simulink model "DrivelineTest"  (R2021a)
settings: Solver=VariableStepAuto  StartTime=0.0  StopTime=10.0  RelTol=1e-3
libraries: sdl_lib x5, fl_lib x3, SimscapeFluids_lib x3, nesl_utility x2
settings Model: Creator=home  LastModifiedBy=home

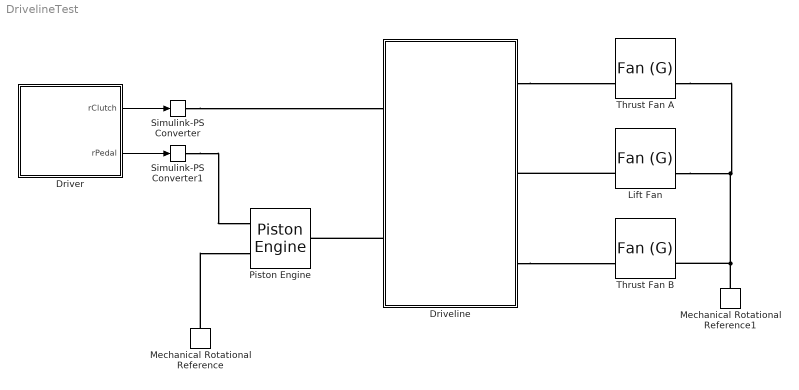
== system DrivelineTest ==
  Driveline : Subsystem
  Driver : Subsystem
  Lift Fan : SimscapeFluids_lib/Gas/Turbomachinery/Fan (G)  fan_spec=fluids.gas.enum.fan_spec.table1D  mech_orientation=simscape.enum.posneg.positive  flow_rate_1D_TLU=[4.7, 5.2, 5.7, 6.1, 6.6] m^3/s  Dp_1D_TLU=[1120, 995.36, 870.94, 746.52, 622.1] Pa  eta_1D_TLU=[.1, .2, .25, .15, .1]  rho_ref_1D=1.2 kg/m^3  omega_ref_1D=910 rpm  omega_Dp_TLU=[450, 500, 550, 600, 650] rpm  flow_rate_Dp_TLU=[.2, .3, .4, .5] m^3/s  Dp_TLU=[675, 650, 560, 420; 830, 800, 695, 520; 1008, 966, 840, 630; 1200, 1150, 1000, 750; 1370, 1300, 1250, 1000] Pa  eta_Dp_TLU=[.22, .23, .25, .24; .38, .39, .4, .34; .58, .6, .62, .6; .81, .82, .84, .8; .88, .91, .95, .9]  omega_flow_TLU=[1800, 2000, 2400, 2800, 3000] rpm  Dp_flow_TLU=[1 / 8, 1 / 4, 3 / 8, 1 / 2] * 3386.4 Pa  flow_rate_TLU=[.3282, .2965, .2556, .1973; .8254, .71, .5876, .4545; 1.2018, 1.0829, .9083, .7034; 1.5065, 1.4098, 1.2722, .9844; 1.8368, 1.7507, 1.6055, 1.2417] m^3/s  eta_flow_TLU=[.22, .23, .25, .24; .38, .39, .4, .34; .58, .6, .62, .6; .81, .82, .84, .8; .88, .91, .95, .9]  omega_DpMax_TLU=[1800, 2000, 2400, 2800, 3000] rpm  DpMax_TLU=[1 / 8, 1 / 4, 3 / 8, 1 / 2, 5 / 8] * 3386.4 Pa  omega_flow_TLU_=[1800, 2000, 2400, 2800, 3000] rpm  Dp_DpMax_TLU=linspace(0, 1, 7)  flow_rate_TLU_=[.3282, .2965, .2556, .1973, .1799, .1288, .0736; .8254, .71, .5876, .4545, .4157, .2967, .1696; 1.2018, 1.0829, .9083, .7034, .6415, .4584, .2619; 1.5065, 1.4098, 1.2722, .9844, .8991, .6418, .3668; 1.8368, 1.7507, 1.6055, 1.2417, 1.1337, .8098, .464] m^3/s  eta_flow_TLU_=[.22, .23, .25, .26, .27, .275, .28; .38, .39, .4, .41, .42, .425, .43; .48, .5, .52, .54, .55, .54, .53; .4, .42, .44, .46, .48, .45, .44; .42, .43, .45, .47, .49, .46, .44]  rho_ref_2D=1.2 kg/m^3  omega_threshold=1 rpm  area_A=0.01 m^2  area_B=0.01 m^2
      settings: SourceProductBaseCode=SH  InternalSimscapePortConfiguration="{\"Bottom\":[],\"Left\":[{\"id\":\"A\",\"label\":\"A\",\"type\":\"foundation.gas.gas\"},{\"id\":\"C\",\"label\":\"C\",\"type\":\"foundation.mechanical.rotational.rotational\"}],\"Right\":[{\"id\":\"B\",\"label\":\"B\",\"type\":\"foundation.gas.gas\"},{\"id\":\"R\",\"label\":\"R\",\"type\":\"foundation.mechanical.rotational.rotational\"}],\"Top\":[]}"
  Mechanical Rotational Reference : fl_lib/Mechanical/Rotational Elements/Mechanical Rotational Reference
  Mechanical Rotational Reference1 : fl_lib/Mechanical/Rotational Elements/Mechanical Rotational Reference
  Piston Engine : sdl_lib/Engines & Motors/Piston Engine  piston_num=4  theta_offset_vector=[0, 180, 360, -180] deg  bore=.10 m  stroke=.06 m  rod=.1 m  stroke_num=4  parameterization=sdl.enum.piston_parameterization.Angle  angle_vector=[-360, -90, -30, 10, 30, 90, 160, 360] deg  throttle_vector=[0, .3, .8, 1]  velocity_vector=[0, 1000, 6000] rpm  pressure_vector=[0, 3, 20, 50, 20, 10, 8, 0] bar  pressure_matrix=[0, 0, 0, 0; 0, .9, 2.4, 3; 0, 6, 16, 20; 0, 15, 40, 50; 0, 6, 16, 20; 0, 3, 8, 10; 0, 2.4, 6.4, 8; 0, 0, 0, 0] bar  pressure_matrix_3D=cat(3, [0, 0, 0, 0; 0, .9, 2.4, 3; 0, 6, 16, 20; 0, 15, 40, 50; 0, 6, 16, 20; 0, 3, 8, 10; 0, 2.4, 6.4, 8; 0, 0, 0, 0], [0, 0, 0, 0; 0, .9, 2.4, 3; 0, 6, 16, 20; 0, 15, 40, 50; 0, 6, 16, 20; 0, 3, 8, 10; 0, 2.4, 6.4, 8; 0, 0, 0, 0], [0, 0, 0, 0; 0, .9, 2.4, 3; 0, 6, 16, 20; 0, 15, 40, 50; 0, 6, 16, 20; 0, 3, 8, 10; 0, 2.4, 6.4, 8; 0, 0, 0, 0]) bar  shaft_dynamics=sdl.enum.shaft_dynamics.On  stiffness=1e6 N*m/rad  damping=1000 N*m/(rad/s)  inertia=.02 kg*m^2  initial_deflection=0 deg  initial_velocity=0 rpm  mu_visc=[0, 0] N*m/(rad/s)  theta_init=90 deg  fc_model=sdl.enum.fuel_consumption_model.FuelOff  fc_per_rev=25 mg/rev  fc_w_tab=[1000, 2000, 3000, 4000, 5000, 6000] rpm  fc_trq_tab=[0, 80, 160, 200, 240, 320, 360, 400] N*m  fc_tab=[.5, .9, 1.4, 1.6, 1.9, 2.7, 3.4, 4.4; 1, 1.7, 2.7, 3.1, 3.6, 5, 6, 7.4; 1.4, 2.7, 4, 4.8, 5.6, 7.5, 8.5, 10.5; 2, 3.6, 5.8, 6.7, 8, 10.4, 11.7, 13.3; 2.5, 4.8, 7.9, 9.4, 10.8, 14, 16.2, 18.6; 3.1, 6, 10.3, 11.9, 13.8, 18.4, 22, 26.5] g/s  bmep_tab=[0, 250, 500, 625, 750, 1000, 1150, 1250] kPa  bsfc_tab=[410, 380, 300, 280, 270, 290, 320, 380; 410, 370, 290, 270, 260, 270, 285, 320; 415, 380, 290, 275, 265, 270, 270, 300; 420, 390, 310, 290, 285, 280, 280, 285; 430, 410, 340, 320, 310, 300, 310, 320; 450, 430, 370, 340, 330, 330, 350, 380] g/hr/kW  fc_interp_method=simscape.enum.interpolation.linear
      settings: SourceProductBaseCode=LD  InternalSimscapePortConfiguration="{\"Bottom\":[],\"Left\":[{\"id\":\"T\",\"label\":\"T\",\"type\":\"input\"},{\"id\":\"B\",\"label\":\"B\",\"type\":\"foundation.mechanical.rotational.rotational\"}],\"Right\":[{\"id\":\"F\",\"label\":\"F\",\"type\":\"foundation.mechanical.rotational.rotational\"}],\"Top\":[]}"
  Simulink-PS Converter : nesl_utility/Simulink-PS Converter  PhysicalDomain=network_engine_domain  SubClassName=ps_input  LeftPortType=input  RightPortType=output  PseudoPeriodic=off  Frequencies=[]  NoiseDistribution=none  NoiseParameters=[]  Unit=1  AffineConversion=off  FilteringAndDerivatives=provide  SimscapeFilterOrder=1  InputFilterTimeConstant=0.001  UdotUserProvided=0
      settings: SourceProductBaseCode=PW,SS
  Simulink-PS Converter1 : nesl_utility/Simulink-PS Converter  PhysicalDomain=network_engine_domain  SubClassName=ps_input  LeftPortType=input  RightPortType=output  PseudoPeriodic=off  Frequencies=[]  NoiseDistribution=none  NoiseParameters=[]  Unit=1  AffineConversion=off  FilteringAndDerivatives=provide  SimscapeFilterOrder=1  InputFilterTimeConstant=0.001  UdotUserProvided=0
      settings: SourceProductBaseCode=PW,SS
  Thrust Fan A : SimscapeFluids_lib/Gas/Turbomachinery/Fan (G)  fan_spec=fluids.gas.enum.fan_spec.table1D  mech_orientation=simscape.enum.posneg.positive  flow_rate_1D_TLU=[4.7, 5.2, 5.7, 6.1, 6.6] m^3/s  Dp_1D_TLU=[1120, 995.36, 870.94, 746.52, 622.1] Pa  eta_1D_TLU=[.1, .2, .25, .15, .1]  rho_ref_1D=1.2 kg/m^3  omega_ref_1D=910 rpm  omega_Dp_TLU=[450, 500, 550, 600, 650] rpm  flow_rate_Dp_TLU=[.2, .3, .4, .5] m^3/s  Dp_TLU=[675, 650, 560, 420; 830, 800, 695, 520; 1008, 966, 840, 630; 1200, 1150, 1000, 750; 1370, 1300, 1250, 1000] Pa  eta_Dp_TLU=[.22, .23, .25, .24; .38, .39, .4, .34; .58, .6, .62, .6; .81, .82, .84, .8; .88, .91, .95, .9]  omega_flow_TLU=[1800, 2000, 2400, 2800, 3000] rpm  Dp_flow_TLU=[1 / 8, 1 / 4, 3 / 8, 1 / 2] * 3386.4 Pa  flow_rate_TLU=[.3282, .2965, .2556, .1973; .8254, .71, .5876, .4545; 1.2018, 1.0829, .9083, .7034; 1.5065, 1.4098, 1.2722, .9844; 1.8368, 1.7507, 1.6055, 1.2417] m^3/s  eta_flow_TLU=[.22, .23, .25, .24; .38, .39, .4, .34; .58, .6, .62, .6; .81, .82, .84, .8; .88, .91, .95, .9]  omega_DpMax_TLU=[1800, 2000, 2400, 2800, 3000] rpm  DpMax_TLU=[1 / 8, 1 / 4, 3 / 8, 1 / 2, 5 / 8] * 3386.4 Pa  omega_flow_TLU_=[1800, 2000, 2400, 2800, 3000] rpm  Dp_DpMax_TLU=linspace(0, 1, 7)  flow_rate_TLU_=[.3282, .2965, .2556, .1973, .1799, .1288, .0736; .8254, .71, .5876, .4545, .4157, .2967, .1696; 1.2018, 1.0829, .9083, .7034, .6415, .4584, .2619; 1.5065, 1.4098, 1.2722, .9844, .8991, .6418, .3668; 1.8368, 1.7507, 1.6055, 1.2417, 1.1337, .8098, .464] m^3/s  eta_flow_TLU_=[.22, .23, .25, .26, .27, .275, .28; .38, .39, .4, .41, .42, .425, .43; .48, .5, .52, .54, .55, .54, .53; .4, .42, .44, .46, .48, .45, .44; .42, .43, .45, .47, .49, .46, .44]  rho_ref_2D=1.2 kg/m^3  omega_threshold=1 rpm  area_A=0.01 m^2  area_B=0.01 m^2
      settings: SourceProductBaseCode=SH  InternalSimscapePortConfiguration="{\"Bottom\":[],\"Left\":[{\"id\":\"A\",\"label\":\"A\",\"type\":\"foundation.gas.gas\"},{\"id\":\"C\",\"label\":\"C\",\"type\":\"foundation.mechanical.rotational.rotational\"}],\"Right\":[{\"id\":\"B\",\"label\":\"B\",\"type\":\"foundation.gas.gas\"},{\"id\":\"R\",\"label\":\"R\",\"type\":\"foundation.mechanical.rotational.rotational\"}],\"Top\":[]}"
  Thrust Fan B : SimscapeFluids_lib/Gas/Turbomachinery/Fan (G)  fan_spec=fluids.gas.enum.fan_spec.table1D  mech_orientation=simscape.enum.posneg.positive  flow_rate_1D_TLU=[4.7, 5.2, 5.7, 6.1, 6.6] m^3/s  Dp_1D_TLU=[1120, 995.36, 870.94, 746.52, 622.1] Pa  eta_1D_TLU=[.1, .2, .25, .15, .1]  rho_ref_1D=1.2 kg/m^3  omega_ref_1D=910 rpm  omega_Dp_TLU=[450, 500, 550, 600, 650] rpm  flow_rate_Dp_TLU=[.2, .3, .4, .5] m^3/s  Dp_TLU=[675, 650, 560, 420; 830, 800, 695, 520; 1008, 966, 840, 630; 1200, 1150, 1000, 750; 1370, 1300, 1250, 1000] Pa  eta_Dp_TLU=[.22, .23, .25, .24; .38, .39, .4, .34; .58, .6, .62, .6; .81, .82, .84, .8; .88, .91, .95, .9]  omega_flow_TLU=[1800, 2000, 2400, 2800, 3000] rpm  Dp_flow_TLU=[1 / 8, 1 / 4, 3 / 8, 1 / 2] * 3386.4 Pa  flow_rate_TLU=[.3282, .2965, .2556, .1973; .8254, .71, .5876, .4545; 1.2018, 1.0829, .9083, .7034; 1.5065, 1.4098, 1.2722, .9844; 1.8368, 1.7507, 1.6055, 1.2417] m^3/s  eta_flow_TLU=[.22, .23, .25, .24; .38, .39, .4, .34; .58, .6, .62, .6; .81, .82, .84, .8; .88, .91, .95, .9]  omega_DpMax_TLU=[1800, 2000, 2400, 2800, 3000] rpm  DpMax_TLU=[1 / 8, 1 / 4, 3 / 8, 1 / 2, 5 / 8] * 3386.4 Pa  omega_flow_TLU_=[1800, 2000, 2400, 2800, 3000] rpm  Dp_DpMax_TLU=linspace(0, 1, 7)  flow_rate_TLU_=[.3282, .2965, .2556, .1973, .1799, .1288, .0736; .8254, .71, .5876, .4545, .4157, .2967, .1696; 1.2018, 1.0829, .9083, .7034, .6415, .4584, .2619; 1.5065, 1.4098, 1.2722, .9844, .8991, .6418, .3668; 1.8368, 1.7507, 1.6055, 1.2417, 1.1337, .8098, .464] m^3/s  eta_flow_TLU_=[.22, .23, .25, .26, .27, .275, .28; .38, .39, .4, .41, .42, .425, .43; .48, .5, .52, .54, .55, .54, .53; .4, .42, .44, .46, .48, .45, .44; .42, .43, .45, .47, .49, .46, .44]  rho_ref_2D=1.2 kg/m^3  omega_threshold=1 rpm  area_A=0.01 m^2  area_B=0.01 m^2
      settings: SourceProductBaseCode=SH  InternalSimscapePortConfiguration="{\"Bottom\":[],\"Left\":[{\"id\":\"A\",\"label\":\"A\",\"type\":\"foundation.gas.gas\"},{\"id\":\"C\",\"label\":\"C\",\"type\":\"foundation.mechanical.rotational.rotational\"}],\"Right\":[{\"id\":\"B\",\"label\":\"B\",\"type\":\"foundation.gas.gas\"},{\"id\":\"R\",\"label\":\"R\",\"type\":\"foundation.mechanical.rotational.rotational\"}],\"Top\":[]}"
  wires:
  Driver/1(rClutch) -> Simulink-PS Converter/1
  Driver/2(rPedal) -> Simulink-PS Converter1/1
  connections:
  Mechanical Rotational Reference/LConn1 -- Piston Engine/LConn2
  Mechanical Rotational Reference1/LConn1 -- Thrust Fan A/RConn2 -- Lift Fan/RConn2 -- Thrust Fan B/RConn2
  Driveline/RConn1 -- Thrust Fan A/LConn2
  Lift Fan/LConn2 -- Driveline/RConn2
  Driveline/LConn2 -- Piston Engine/RConn1
  Driveline/RConn3 -- Thrust Fan B/LConn2
  Simulink-PS Converter/RConn1 -- Driveline/LConn1
  Simulink-PS Converter1/RConn1 -- Piston Engine/LConn1

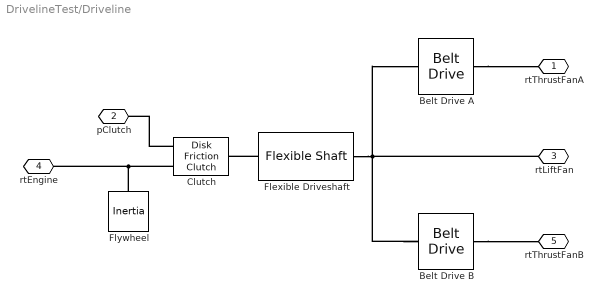
== system DrivelineTest/Driveline ==
  Belt Drive A : sdl_lib/Couplings & Drives/Belt Drive  drive_type=sdl.enum.wrap_configuration.open  belt_type=sdl.enum.belt_type.ideal  sheave_ang=30 deg  num_belts=1  model_f_c=sdl.enum.model_centrifugal.off  linear_density=0.6 kg/m  model_compliance=sdl.enum.compliance.on  stiffness=1e4 N/m  damping=1e3 N/(m/s)  tension=100 N  breakable=sdl.enum.max_tension.off  F_max=1e5 N  r_pulley_A=.15 m  r_pulley_B=.30 m  b_pulley_A=0 N*m/(rad/s)  b_pulley_B=0.001 N*m/(rad/s)  model_inertia_A=sdl.enum.model_inertia.off  model_inertia_B=sdl.enum.model_inertia.off  pulley_inertia_A=0.01 kg*m^2  pulley_inertia_B=0.03 kg*m^2  initial_velocity_A=0 rad/s  initial_velocity_B=0 rad/s  mu=0.5  wrap_parameterization=sdl.enum.wrap_parameterization.centers  d_centers=0.5 m  phi_wrap_A=145 deg  phi_wrap_B=215 deg  v_thr=0.001 m/s
      settings: SourceProductBaseCode=LD  InternalSimscapePortConfiguration="{\"Bottom\":[],\"Left\":[{\"id\":\"A\",\"label\":\"A\",\"type\":\"foundation.mechanical.rotational.rotational\"}],\"Right\":[{\"id\":\"B\",\"label\":\"B\",\"type\":\"foundation.mechanical.rotational.rotational\"}],\"Top\":[]}"
  Belt Drive B : sdl_lib/Couplings & Drives/Belt Drive  drive_type=sdl.enum.wrap_configuration.open  belt_type=sdl.enum.belt_type.ideal  sheave_ang=30 deg  num_belts=1  model_f_c=sdl.enum.model_centrifugal.off  linear_density=0.6 kg/m  model_compliance=sdl.enum.compliance.on  stiffness=1e4 N/m  damping=1e3 N/(m/s)  tension=100 N  breakable=sdl.enum.max_tension.off  F_max=1e5 N  r_pulley_A=.15 m  r_pulley_B=.30 m  b_pulley_A=0 N*m/(rad/s)  b_pulley_B=0.001 N*m/(rad/s)  model_inertia_A=sdl.enum.model_inertia.off  model_inertia_B=sdl.enum.model_inertia.off  pulley_inertia_A=0.01 kg*m^2  pulley_inertia_B=0.03 kg*m^2  initial_velocity_A=0 rad/s  initial_velocity_B=0 rad/s  mu=0.5  wrap_parameterization=sdl.enum.wrap_parameterization.centers  d_centers=0.5 m  phi_wrap_A=145 deg  phi_wrap_B=215 deg  v_thr=0.001 m/s
      settings: SourceProductBaseCode=LD  InternalSimscapePortConfiguration="{\"Bottom\":[],\"Left\":[{\"id\":\"A\",\"label\":\"A\",\"type\":\"foundation.mechanical.rotational.rotational\"}],\"Right\":[{\"id\":\"B\",\"label\":\"B\",\"type\":\"foundation.mechanical.rotational.rotational\"}],\"Top\":[]}"
  Clutch : sdl_lib/Clutches/Disk Friction Clutch  geometry_model=sdl.enum.friction_geometry.radius  r_eff=130 mm  d_o=150 mm  d_i=100 mm  nS=4  piston_area=0.001 m^2  unidirectional=sdl.enum.directionality.bidirectional  friction_model=sdl.enum.friction_model_TLU_thermal.fixed  mu_w_vector=[0, 100, 1000] rad/s  temperature_TLU=[280, 300, 320] K  mu_static=0.35  mu_static_vector=[.4, .38, .36]  mu_coulomb=0.3  mu_coulomb_vector=[.3, .22, .19]  mu_coulomb_temp_vector=[.3, .28, .25]  mu_coulomb_matrix=[.34, .32, .3; .3, .28, .25; .25, .2, .15]  mu_interp_method=simscape.enum.interpolation.linear  mu_extrap_method=simscape.enum.extrapolation.linear  d_f=1  w_tol=0.001 rad/s  pressure_min=100 Pa  mu_visc=0 N*m/(rad/s)  initial_state_locked=sdl.enum.initial_lock.unlocked  enable_faults=simscape.enum.onoff.off  fault_type=sdl.enum.clutchFault.lock  external_fault=simscape.enum.onoff.off  temporal_fault=simscape.enum.onoff.off  fault_time=5 s  report_fault=simscape.enum.assert.action.none  thermal_mass=50 kJ/K  T_init=300 K
      settings: SourceProductBaseCode=LD  InternalSimscapePortConfiguration="{\"Bottom\":[],\"Left\":[{\"id\":\"P\",\"label\":\"P\",\"type\":\"input\"},{\"id\":\"B\",\"label\":\"B\",\"type\":\"foundation.mechanical.rotational.rotational\"}],\"Right\":[{\"id\":\"F\",\"label\":\"F\",\"type\":\"foundation.mechanical.rotational.rotational\"}],\"Top\":[]}"
  Flexible Driveshaft : sdl_lib/Couplings & Drives/Flexible Shaft  modelTransverse=simscape.enum.onoff.off  n_segments=1  parameterization=sdl.enum.shaftParameterization.StiffnessInertia  length=1 m  lengths=[1, .5, .25] m  shaft_stiffness=2e5 N*m/rad  shaft_inertia=0.02 kg*m^2  shaft_stiffnesses=[400000, 200000, 100000] N*m/rad  shaft_inertias=[.025, .02, .015] kg*m^2  eiIN=5e5 m^4*Pa  rhoaIN=19 kg/m  eiINs=[600000, 500000, 400000] m^4*Pa  rhoaINs=[20, 19, 18] kg/m  density=7.8e3 kg/m^3  shear_modulus=7.93e9 Pa  elastic_modulus=200e9 Pa  shaft_construction=sdl.enum.shaftConstruction.solid  diameter_outer=0.075 m  diameter_inner=0.05 m  diameter_outers=[.085, .075, .065] m  diameter_inners=[.055, .05, .045] m  damping_ratio=0.01  mu_visc_BF=[0, 0] N*m/(rad/s)  mu_visc=[0, 0] N*m/(rad/s)  initial_deflection=0 rad  initial_velocity=0 rpm  num_supports=sdl.enum.num_supports.two  z_support=[0, 1] m  boundaryB1=sdl.enum.shaftSupport.clamp  DrotB1_row=[1000, 1000] N*m/(rad/s)  DtransB1_row=[20000, -44000, -44000, 350000] N/(m/s)  DtransB1_w_mat=[20000, -44000, -44000, 350000; 10000, -25000, -25000, 140000; 5000, -10000, -10000, 20000] N/(m/s)  KrotB1_row=[10000, 10000] N*m/rad  KtransB1_row=[1000000, -200000, -300000, 5000000] N/m  KtransB1_w_mat=[1000000, -600000, -3500000, 8000000; 1000000, -200000, -3000000, 5000000; 1000000, -50000, -2500000, 3000000] N/m  boundaryI1=sdl.enum.shaftSupport.clamp  DrotI1_row=[1000, 1000] N*m/(rad/s)  DtransI1_row=[20000, -44000, -44000, 350000] N/(m/s)  DtransI1_w_mat=[20000, -44000, -44000, 350000; 10000, -25000, -25000, 140000; 5000, -10000, -10000, 20000] N/(m/s)  KrotI1_row=[10000, 10000] N*m/rad  KtransI1_row=[1000000, -200000, -300000, 5000000] N/m  KtransI1_w_mat=[1000000, -600000, -3500000, 8000000; 1000000, -200000, -3000000, 5000000; 1000000, -50000, -2500000, 3000000] N/m  boundaryI2=sdl.enum.shaftSupport.clamp  DrotI2_row=[1000, 1000] N*m/(rad/s)  DtransI2_row=[20000, -44000, -44000, 350000] N/(m/s)  DtransI2_w_mat=[20000, -44000, -44000, 350000; 10000, -25000, -25000, 140000; 5000, -10000, -10000, 20000] N/(m/s)  KrotI2_row=[10000, 10000] N*m/rad  KtransI2_row=[1000000, -200000, -300000, 5000000] N/m  KtransI2_w_mat=[1000000, -600000, -3500000, 8000000; 1000000, -200000, -3000000, 5000000; 1000000, -50000, -2500000, 3000000] N/m  boundaryF1=sdl.enum.shaftSupport.clamp  DrotF1_row=[1000, 1000] N*m/(rad/s)  DtransF1_row=[20000, -44000, -44000, 350000] N/(m/s)  DtransF1_w_mat=[20000, -44000, -44000, 350000; 10000, -25000, -25000, 140000; 5000, -10000, -10000, 20000] N/(m/s)  KrotF1_row=[10000, 10000] N*m/rad  KtransF1_row=[1000000, -200000, -300000, 5000000] N/m  KtransF1_w_mat=[1000000, -600000, -3500000, 8000000; 1000000, -200000, -3000000, 5000000; 1000000, -50000, -2500000, 3000000] N/m  bearing_speed=[200, 500, 1500] rpm  alpha=10 1/s  beta=1e-8 s  noDisk=sdl.enum.shaftDisks.none  zDisk=0.5 m  mDiskIN=2 kg  IdDiskIN=0.025 kg*m^2  IpDiskIN=0.050 kg*m^2  offsetMR=[.01, .01] m*kg  offsetMassLocation=[.33, .67] m  offsetMR_initialAngleIN=[0, pi] rad  AnalysisMethod=sdl.enum.bendingAnalysisMethod.LumpedMass  ModeInputMethod=sdl.enum.modeInputMethod.SimscapeDetermined  numModesIn=6  mode_speed_dependency=sdl.enum.mode_speed_dependency.Static  OmegaNom=5000 rpm  wMax=1e8 rpm  dz=0.01 m  userMode_w=[280, 644, 615, 1285] rad/s  userMode_w_mat=[257, 780, 580, 1560; 280, 644, 615, 1285; 294, 513, 636, 1020] rad/s  userMode_z=[0, .1, .2, .3, .4, .5, .6, .7, .8, .9, 1] m  userMode_shapeX=[.1648, .0086, -.2759, .0162; .1671, .0093, -.2231, .0133; .1691, .01, -.1689, .0102; .1707, .0105, -.1135, .007; .1717, .0108, -.057, .0035; .1721, .0109, 0, 0; .1717, .0108, .057, -.0035; .1707, .0105, .1135, -.007; .1691, .01, .1689, -.0102; .1671, .0093, .2231, -.0133; .1648, .0086, .2759, -.0162]  userMode_shapeX_mat=cat(3, [.1842, .0134, -.3072, .0272; .1863, .0152, -.2482, .0226; .1882, .0169, -.1878, .0176; .1897, .0182, -.1261, .0121; .1906, .019, -.0634, .0062; .191, .0193, 0, 0; .1906, .019, .0634, -.0062; .1897, .0182, .1261, -.0121; .1882, .0169, .1878, -.0176; .1863, .0152, .2482, -.0226; .1842, .0134, .3072, -.0272], [.1648, .0086, -.2759, .0162; .1671, .0093, -.2231, .0133; .1691, .01, -.1689, .0102; .1707, .0105, -.1135, .007; .1717, .0108, -.057, .0035; .1721, .0109, 0, 0; .1717, .0108, .057, -.0035; .1707, .0105, .1135, -.007; .1691, .01, .1689, -.0102; .1671, .0093, .2231, -.0133; .1648, .0086, .2759, -.0162], [.1291, .0046, -.2166, .0082; .131, .0048, -.1751, .0067; .1327, .005, -.1327, .0051; .1341, .0052, -.0891, .0035; .135, .0053, -.0448, .0017; .1353, .0053, 0, 0; .135, .0053, .0448, -.0017; .1341, .0052, .0891, -.0035; .1327, .005, .1327, -.0051; .131, .0048, .1751, -.0067; .1291, .0046, .2166, -.0082])  userMode_shapeY=[.1193, -.1784, -.1997, -.3348; .1209, -.1933, -.1615, -.2751; .1224, -.2068, -.1223, -.2119; .1235, -.2176, -.0821, -.1445; .1243, -.2245, -.0413, -.0734; .1246, -.2269, 0, 0; .1243, -.2245, .0413, .0734; .1235, -.2176, .0821, .1445; .1224, -.2068, .1223, .2119; .1209, -.1933, .1615, .2751; .1193, -.1784, .1997, .3348]  userMode_shapeY_mat=cat(3, [.0885, -.1625, -.1475, -.3301; .0895, -.1847, -.1192, -.2745; .0904, -.2048, -.0902, -.2141; .0911, -.2209, -.0606, -.1475; .0916, -.2313, -.0304, -.0754; .0917, -.2349, 0, 0; .0916, -.2313, .0304, .0754; .0911, -.2209, .0606, .1475; .0904, -.2048, .0902, .2141; .0895, -.1847, .1192, .2745; .0885, -.1625, .1475, .3301], [.1193, -.1784, -.1997, -.3348; .1209, -.1933, -.1615, -.2751; .1224, -.2068, -.1223, -.2119; .1235, -.2176, -.0821, -.1445; .1243, -.2245, -.0413, -.0734; .1246, -.2269, 0, 0; .1243, -.2245, .0413, .0734; .1235, -.2176, .0821, .1445; .1224, -.2068, .1223, .2119; .1209, -.1933, .1615, .2751; .1193, -.1784, .1997, .3348], [.1566, -.1901, -.2628, -.3377; .1589, -.1994, -.2125, -.2753; .161, -.2079, -.1609, -.2103; .1627, -.2146, -.1081, -.1424; .1638, -.219, -.0544, -.0719; .1642, -.2205, 0, 0; .1638, -.219, .0544, .0719; .1627, -.2146, .1081, .1424; .161, -.2079, .1609, .2103; .1589, -.1994, .2125, .2753; .1566, -.1901, .2628, .3377])
      settings: SourceProductBaseCode=LD  InternalSimscapePortConfiguration="{\"Bottom\":[],\"Left\":[{\"id\":\"B\",\"label\":\"B\",\"type\":\"foundation.mechanical.rotational.rotational\"}],\"Right\":[{\"id\":\"F\",\"label\":\"F\",\"type\":\"foundation.mechanical.rotational.rotational\"}],\"Top\":[]}"
  Flywheel : fl_lib/Mechanical/Rotational Elements/Inertia  inertia=0.01 kg*m^2  num_ports=foundation.enum.numPorts2.one  w_specify=off  w_priority=High  w=0 rad/s  w_nominal_specify=off  w_nominal_unit=rad/s  w_nominal_value=1  t_specify=off  t_priority=None  t=0 N*m  t_nominal_specify=off  t_nominal_unit=N*m  t_nominal_value=1
  rtThrustFanA : PMIOPort  Side=Right
  pClutch : PMIOPort  Port=2  Side=Left
  rtLiftFan : PMIOPort  Port=3  Side=Right
  rtEngine : PMIOPort  Port=4  Side=Left
  rtThrustFanB : PMIOPort  Port=5  Side=Right
  connections:
  Flexible Driveshaft/RConn1 -- Belt Drive B/LConn1 -- rtLiftFan/RConn1 -- Belt Drive A/LConn1
  Belt Drive B/RConn1 -- rtThrustFanB/RConn1
  Clutch/LConn2 -- rtEngine/RConn1 -- Flywheel/LConn1
  Flexible Driveshaft/LConn1 -- Clutch/RConn1
  Belt Drive A/RConn1 -- rtThrustFanA/RConn1
  Clutch/LConn1 -- pClutch/RConn1

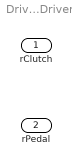
== system DrivelineTest/Driver ==
  rClutch : Outport
  rPedal : Outport  Port=2
